simulink model "qam16"  (R2013b)
settings: Solver=FixedStepDiscrete  StartTime=0.0  StopTime=0.2e-3  RelTol=1e-3
InitFcn:
  | Fs=20e6;
libraries: commfilt2 x3, commrandsrc2 x2, commdigbbndam3 x2
settings Model: Creator=josulliv  LastModifiedBy=DPu1

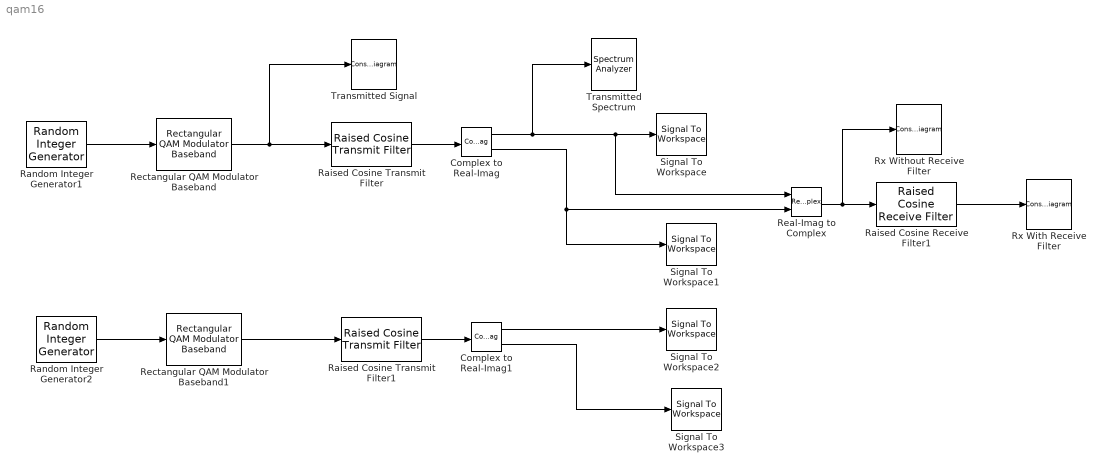
== system qam16 ==
  Complex to Real-Imag : ComplexToRealImag
  Complex to Real-Imag1 : ComplexToRealImag
  Raised Cosine Receive Filter1 : commfilt2/Raised Cosine Receive Filter  filtType=Square root  N=8  filtSpan=6  currentFiltSpan=2*(3)  D=(2*(3))/2  R=0.3  sampMode=Mute  saveAsFlag=0  rateMode=Downsampling  downFactor=8  downOffset=0  framing=Enforce single-rate processing  InputProcessing=Columns as channels (frame based)  checkGain=Normalized  filterGain=1  checkCoeff=off  variableName=rcRxFilt1  launchFVT=off  roundingMode=Floor  overflowMode=off
  Raised Cosine Transmit Filter : commfilt2/Raised Cosine Transmit Filter  filtType=Square root  filtSpan=6  currentFiltSpan=6  D=(6)/2  R=0.3  sampMode=Mute  saveAsFlag=0  N=8  framing=Enforce single-rate processing  InputProcessing=Columns as channels (frame based)  checkGain=Normalized  filterGain=1  checkCoeff=off  variableName=rcTxFilt1  launchFVT=off  roundingMode=Floor  overflowMode=off
  Raised Cosine Transmit Filter1 : commfilt2/Raised Cosine Transmit Filter  filtType=Square root  filtSpan=6  currentFiltSpan=6  D=(6)/2  R=0.3  sampMode=Mute  saveAsFlag=0  N=8  framing=Enforce single-rate processing  InputProcessing=Columns as channels (frame based)  checkGain=Normalized  filterGain=1  checkCoeff=off  variableName=rcTxFilt1  launchFVT=off  roundingMode=Floor  overflowMode=off
  Random Integer Generator1 : commrandsrc2/Random Integer Generator  mul=16  seed=37  Ts=1/Fs  frameBased=on  sampPerFrame=100  orient=off  outDataType=double
  Random Integer Generator2 : commrandsrc2/Random Integer Generator  mul=16  seed=73  Ts=1/Fs  frameBased=on  sampPerFrame=100  orient=off  outDataType=double
  Real-Imag to Complex : RealImagToComplex
  Rectangular QAM Modulator Baseband : commdigbbndam3/Rectangular QAM Modulator Baseband  M=16  InType=Integer  Enc=Binary  Mapping=[0:15]  PowType=Average Power  MinDist=2  AvgPow=1  PeakPow=1  Ph=0  outDtype=double  outWordLen=16  outUDDataType=sfix(16)  outFracLenMode=Best precision  outFracLen=15
  Rectangular QAM Modulator Baseband1 : commdigbbndam3/Rectangular QAM Modulator Baseband  M=16  InType=Integer  Enc=Binary  Mapping=[0:15]  PowType=Average Power  MinDist=2  AvgPow=1  PeakPow=1  Ph=0  outDtype=double  outWordLen=16  outUDDataType=sfix(16)  outFracLenMode=Best precision  outFracLen=15
  Rx With Receive Filter : ConstellationDiagram  Tag=ScatterPlot
      settings: CopyFcn=scopeextensions.ScopeBlock.onCoreBlockCopy(gcbh);  DeleteFcn=scopeextensions.ScopeBlock.callback(gcbh, 'onBlockDelete');  PreSaveFcn=scopeextensions.ScopeBlock.callback(gcbh, 'onModelSave');  NameChangeFcn=scopeextensions.ScopeBlock.callback(gcbh, 'onBlockRename');  DestroyFcn=scopeextensions.ScopeBlock.onBlockDestroy(gcbh)  CloseFcn=scopeextensions.ScopeBlock.callback(gcbh, 'onBlockClose');  PreDeleteFcn=scopeextensions.ScopeBlock.callback(gcbh, 'onBlockPreDelete');
  Rx Without Receive Filter : ConstellationDiagram  Tag=ScatterPlot
      settings: CopyFcn=scopeextensions.ScopeBlock.onCoreBlockCopy(gcbh);  DeleteFcn=scopeextensions.ScopeBlock.callback(gcbh, 'onBlockDelete');  PreSaveFcn=scopeextensions.ScopeBlock.callback(gcbh, 'onModelSave');  NameChangeFcn=scopeextensions.ScopeBlock.callback(gcbh, 'onBlockRename');  DestroyFcn=scopeextensions.ScopeBlock.onBlockDestroy(gcbh)  CloseFcn=scopeextensions.ScopeBlock.callback(gcbh, 'onBlockClose');  PreDeleteFcn=scopeextensions.ScopeBlock.callback(gcbh, 'onBlockPreDelete');
  Signal To Workspace : SignalToWorkspace  VariableName=I1
      settings: CopyFcn=dspblkcopystw(gcbh);
  Signal To Workspace1 : SignalToWorkspace  VariableName=Q1
      settings: CopyFcn=dspblkcopystw(gcbh);
  Signal To Workspace2 : SignalToWorkspace  VariableName=I2
      settings: CopyFcn=dspblkcopystw(gcbh);
  Signal To Workspace3 : SignalToWorkspace  VariableName=Q2
      settings: CopyFcn=dspblkcopystw(gcbh);
  Transmitted Signal : ConstellationDiagram  Tag=ScatterPlot
      settings: CopyFcn=scopeextensions.ScopeBlock.onCoreBlockCopy(gcbh);  DeleteFcn=scopeextensions.ScopeBlock.callback(gcbh, 'onBlockDelete');  PreSaveFcn=scopeextensions.ScopeBlock.callback(gcbh, 'onModelSave');  NameChangeFcn=scopeextensions.ScopeBlock.callback(gcbh, 'onBlockRename');  DestroyFcn=scopeextensions.ScopeBlock.onBlockDestroy(gcbh)  CloseFcn=scopeextensions.ScopeBlock.callback(gcbh, 'onBlockClose');  PreDeleteFcn=scopeextensions.ScopeBlock.callback(gcbh, 'onBlockPreDelete');
  Transmitted Spectrum : SpectrumAnalyzer
      settings: CopyFcn=scopeextensions.ScopeBlock.onCoreBlockCopy(gcbh);  DeleteFcn=scopeextensions.ScopeBlock.callback(gcbh, 'onBlockDelete');  PreSaveFcn=scopeextensions.ScopeBlock.callback(gcbh, 'onModelSave');  NameChangeFcn=scopeextensions.ScopeBlock.callback(gcbh, 'onBlockRename');  DestroyFcn=scopeextensions.ScopeBlock.onBlockDestroy(gcbh)  CloseFcn=scopeextensions.ScopeBlock.callback(gcbh, 'onBlockClose');  PreDeleteFcn=scopeextensions.ScopeBlock.callback(gcbh, 'onBlockPreDelete');
  wires:
  Rectangular QAM Modulator Baseband/1 -> Transmitted Signal/1, Raised Cosine Transmit Filter/1
  Complex to Real-Imag/1 -> Transmitted Spectrum/1, Real-Imag to Complex/1, Signal To Workspace/1
  Complex to Real-Imag/2 -> Real-Imag to Complex/2, Signal To Workspace1/1
  Real-Imag to Complex/1 -> Rx Without Receive Filter/1, Raised Cosine Receive Filter1/1
  Raised Cosine Receive Filter1/1 -> Rx With Receive Filter/1
  Random Integer Generator1/1 -> Rectangular QAM Modulator Baseband/1
  Raised Cosine Transmit Filter/1 -> Complex to Real-Imag/1
  Rectangular QAM Modulator Baseband1/1 -> Raised Cosine Transmit Filter1/1
  Complex to Real-Imag1/1 -> Signal To Workspace2/1
  Complex to Real-Imag1/2 -> Signal To Workspace3/1
  Random Integer Generator2/1 -> Rectangular QAM Modulator Baseband1/1
  Raised Cosine Transmit Filter1/1 -> Complex to Real-Imag1/1
